simulink model "Problem9"  (R2020b)
settings: Solver=VariableStepAuto  StartTime=0.0  StopTime=10.0  RelTol=1e-3
InitFcn:
  | data
values from neighbouring files (symbols this model uses):
  Ke = 0.06902    [data.m]
  taue = 151.51*10^-6    (= 0.00015151)    [data.m]
  taum = 0.0161    [data.m]
settings Model: Creator=Acer  LastModifiedBy=Acer

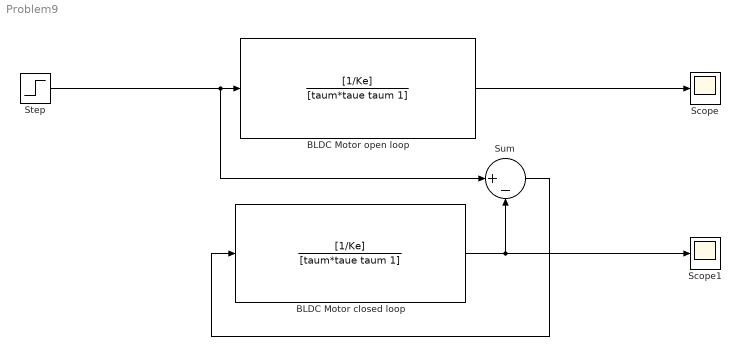
== system Problem9 ==
  BLDC Motor closed loop : TransferFcn  Numerator=[1/Ke]  Denominator=[taum*taue taum 1]
  BLDC Motor open loop : TransferFcn  Numerator=[1/Ke]  Denominator=[taum*taue taum 1]
  Scope : Scope
  Scope1 : Scope
  Step : Step  Time=0  SampleTime=0
  Sum : Sum  Inputs=|+-
  wires:
  Step/1 -> BLDC Motor open loop/1, Sum/1
  Sum/1 -> BLDC Motor closed loop/1
  BLDC Motor closed loop/1 -> Sum/2, Scope1/1
  BLDC Motor open loop/1 -> Scope/1
